simulink model "Demo_init"  (R2022b)
settings: Solver=ode23tb  StartTime=0.0  StopTime=630  RelTol=1e-3
undefined symbols (not defined in the file or in its folder): Azimuth_initial_angle, Elevation_initial_angle, i_gearbox_1, i_gearbox_2, J_azimuth, J_elevation, J_engine, J_gearbox_1, J_gearbox_2, Kku, Km, Kw, L, R
settings Model: Creator=Maxim Kozlov  LastModifiedBy=KozlovM
settings OptimizationCC: ReuseModelBlockBuffer=on

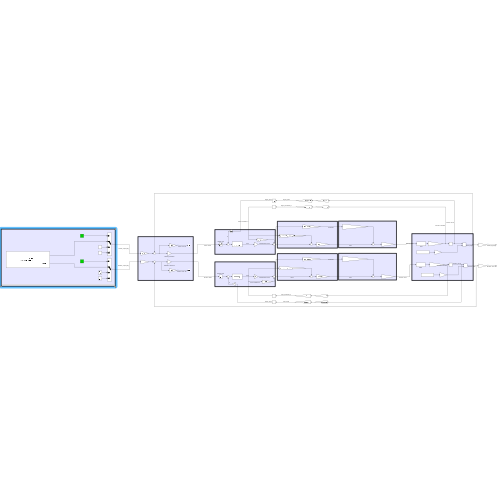
[thumbnail: Simulink's stored preview of the top-level diagram]
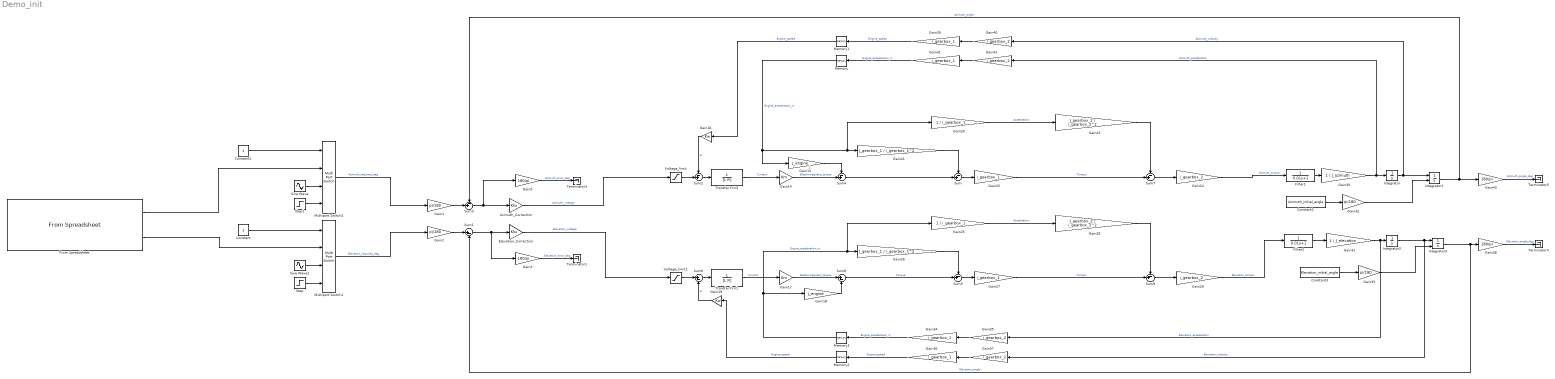
== system Demo_init ==
  note: J
  Azimuth_Correction : Gain  Gain=Kku
  Constant : Constant
  Constant1 : Constant
  Constant2 : Constant  Value=Azimuth_initial_angle
  Constant3 : Constant  Value=Elevation_initial_angle
  Elevation_Correction : Gain  Gain=Kku
  Filter1 : TransferFcn  Denominator=[0.01 1]
  Filter2 : TransferFcn  Denominator=[0.01 1]
  From Spreadsheet : FromSpreadsheet  FileName=.\data\DemoSatelliteData.xlsx  SheetName=International_Space_Station
  Gain{1..2,32..33} (4 alike) : Gain  Gain=pi/180
  Gain14 : Gain  Gain=Km
  Gain15 : Gain  Gain=J_engine
  Gain16 : Gain  Gain=Kw
  Gain17 : Gain  Gain=Km
  Gain18 : Gain  Gain=J_engine
  Gain19 : Gain  Gain=Kw
  Gain20 : Gain  Gain=1 / i_gearbox_1
  Gain21 : Gain  Gain=J_gearbox_1 / i_gearbox_1^2
  Gain{22,27,34,36,39,41} (6 alike) : Gain  Gain=i_gearbox_1
  Gain23 : Gain  Gain=J_gearbox_2 / i_gearbox_2^2
  Gain{24,29,35,37,40,42} (6 alike) : Gain  Gain=i_gearbox_2
  Gain25 : Gain  Gain=1 / i_gearbox_1
  Gain26 : Gain  Gain=J_gearbox_1 / i_gearbox_1^2
  Gain28 : Gain  Gain=J_gearbox_2 / i_gearbox_2^2
  Gain{3,5,38,43} (4 alike) : Gain  Gain=180/pi
  Gain30 : Gain  Gain=1 / J_azimuth
  Gain31 : Gain  Gain=1 / J_elevation
  Integrator : Integrator
  Integrator1 : Integrator  InitialConditionSource=external
  Integrator2 : Integrator
  Integrator3 : Integrator  InitialConditionSource=external
  Memory{,1..3} (4 alike) : Memory
  Multiport Switch1 : MultiPortSwitch  SaturateOnIntegerOverflow=off  InputSameDT=off
  Multiport Switch2 : MultiPortSwitch  SaturateOnIntegerOverflow=off  InputSameDT=off
  Sine Wave : Sin  Amplitude=6  Phase=pi/2  SampleTime=0
  Sine Wave1 : Sin  Amplitude=6  SampleTime=0
  Step : Step  SampleTime=0
  Step1 : Step  SampleTime=0
  Sum{,2..5,7,9} (7 alike) : Sum  Inputs=-+|
  Sum1 : Sum  Inputs=|+-
  Sum6 : Sum  Inputs=|+-
  Sum8 : Sum  Inputs=|+-
  Terminator{1,3..5} (4 alike) : Terminator
  Transfer Fcn1 : TransferFcn  Denominator=[L R]
  Transfer Fcn3 : TransferFcn  Denominator=[L R]
  Voltage_limit : Saturate  UpperLimit=10.8  LowerLimit=-10.8
  Voltage_limit1 : Saturate  UpperLimit=10.8  LowerLimit=-10.8
  wires:
  Gain34/1 -> Memory3/1  "Engine_acceleration_in"
  Gain17/1 -> Sum8/1  "Electromagnetic_torque"
  Constant/1 -> Multiport Switch1/1
  Gain28/1 -> Sum9/1
  Sum/1 -> Gain22/1
  Gain23/1 -> Sum7/1
  Sum7/1 -> Gain24/1
  Sum4/1 -> Sum/2
  Transfer Fcn3/1 -> Gain14/1  "Сurrent"
  Gain20/1 -> Gain23/1  "Acceleration"
  Azimuth_Correction/1 -> Voltage_limit/1  "Azimuth_voltage"
  Gain14/1 -> Sum4/2  "Electromagnetic_torque"
  Gain39/1 -> Memory1/1  "Engine_speed"
  Gain43/1 -> Terminator5/1  "Azimuth_angle_deg"
  Integrator3/1 -> Gain38/1, Sum1/2  "Elevation_angle"
  Gain40/1 -> Gain39/1
  Gain42/1 -> Gain41/1
  Gain21/1 -> Sum/1
  Sine Wave1/1 -> Multiport Switch1/3
  Gain41/1 -> Memory/1  "Engine_acceleration_in"
  Gain36/1 -> Memory2/1  "Engine_speed"
  Gain18/1 -> Sum8/2
  Gain31/1 -> Integrator2/1, Gain35/1  "Elevation_acceleration"
  Gain37/1 -> Gain36/1
  Integrator2/1 -> Integrator3/1, Gain37/1  "Elevation_velocity"
  Gain2/1 -> Sum1/1
  Constant2/1 -> Gain32/1
  Gain24/1 -> Filter1/1  "Azimuth_torque"
  Gain38/1 -> Terminator4/1  "Elevation_angle_deg"
  Gain30/1 -> Gain42/1, Integrator/1  "Azimuth_acceleration"
  Gain32/1 -> Integrator1/2
  Constant3/1 -> Gain33/1
  Multiport Switch1/1 -> Gain2/1  "Elevation_required_deg"
  Sum6/1 -> Transfer Fcn1/1
  Gain5/1 -> Terminator3/1  "Azimuth_error_deg"
  Gain19/1 -> Sum6/2  "E"
  Transfer Fcn1/1 -> Gain17/1  "Сurrent"
  Gain16/1 -> Sum2/1  "E"
  Gain33/1 -> Integrator3/2
  Gain22/1 -> Sum7/2  "Torque"
  Gain26/1 -> Sum5/1
  Voltage_limit1/1 -> Sum6/1
  Sum9/1 -> Gain29/1
  Integrator1/1 -> Gain43/1, Sum3/1  "Azimuth_angle"
  Gain25/1 -> Gain28/1  "Acceleration"
  Sum3/1 -> Gain5/1, Azimuth_Correction/1
  Sum5/1 -> Gain27/1
  Elevation_Correction/1 -> Voltage_limit1/1  "Elevation_voltage"
  Integrator/1 -> Gain40/1, Integrator1/1  "Azimuth_velocity"
  Gain3/1 -> Terminator1/1  "Elevation_error_deg"
  From Spreadsheet/1 -> Multiport Switch2/2
  From Spreadsheet/2 -> Multiport Switch1/2
  Step1/1 -> Multiport Switch2/4
  Gain29/1 -> Filter2/1  "Elevation_torque"
  Voltage_limit/1 -> Sum2/2
  Constant1/1 -> Multiport Switch2/1
  Gain35/1 -> Gain34/1
  Gain1/1 -> Sum3/2
  Multiport Switch2/1 -> Gain1/1  "Azimuth_required_deg"
  Sum2/1 -> Transfer Fcn3/1
  Gain27/1 -> Sum9/2  "Torque"
  Sine Wave/1 -> Multiport Switch2/3
  Sum8/1 -> Sum5/2  "Torque"
  Sum1/1 -> Gain3/1, Elevation_Correction/1
  Step/1 -> Multiport Switch1/4
  Gain15/1 -> Sum4/1
  Memory/1 -> Gain20/1, Gain21/1, Gain15/1  "Engine_acceleration_in"
  Memory1/1 -> Gain16/1  "Engine_speed"
  Memory2/1 -> Gain19/1  "Engine_speed"
  Memory3/1 -> Gain26/1, Gain25/1, Gain18/1  "Engine_acceleration_in"
  Filter1/1 -> Gain30/1
  Filter2/1 -> Gain31/1
